simulink model "TGB_V0000"  (R2016b)
settings: Solver=VariableStepAuto  StartTime=0.0  StopTime=350  RelTol=1e-3
values from neighbouring files (symbols this model uses):
  h = 30    [AutoPID.m]
  K = data.Data(len)/100    [AutoPID.m]
  Kp = 0.6*Kc    (= 0.48762365543)    [AutoPID.m]
  Malha = 1    [AutoPID.m]
  N = 1    [AutoPID.m]
  T = (10*wn)/2*pi    [AutoPID.m]
  T_PID = 1    [AutoPID.m]
  tau = (3/2)*(t2-t1)    [AutoPID.m]
  Td = Tc*0.125    (= 41.8060200669)    [AutoPID.m]
  theta = t2-tau    [AutoPID.m]
  Ti = Tc*0.5    (= 167.224080268)    [AutoPID.m]
  TypeControler = 1    [AutoPID.m]
  TypeOutput = 1    [AutoPID.m]
undefined symbols (not defined in the file or in its folder): DiscIntNeverNeededParam
libraries: simulink x2
settings Model: Creator=Workstation - LFC  LastModifiedBy=Gpiaia
settings DataIOCC: SaveOutput=off  SaveTime=off
settings OptimizationCC: DefaultParameterBehavior=Inlined  UseDivisionForNetSlopeComputation=on  UseFloatMulNetSlope=on  InlineInvariantSignals=on  PassReuseOutputArgsAs=Individual arguments  ZeroExternalMemoryAtStartup=off  ZeroInternalMemoryAtStartup=off  NoFixptDivByZeroProtection=on  EfficientFloat2IntCast=on  LifeSpan=1
settings DebuggingCC: ParameterTunabilityLossMsg=error  SFExecutionAtInitializationDiag=none
settings HardwareCC: ProdBitPerLong=64  ProdHWDeviceType=Intel->x86-64 (Linux 64)
settings RTWCC: SystemTargetFile=ert.tlc  TemplateMakefile=ert_default_tmf  Description=Embedded Coder  GenerateReport=on  IncludeHyperlinkInReport=on  LaunchReport=on  GenerateTraceInfo=on  GenerateTraceReport=on  GenerateTraceReportSl=on  GenerateTraceReportSf=on  GenerateTraceReportEml=on  GenerateCodeMetricsReport=on
settings CodeAppCC: ForceParamTrailComments=on  IgnoreCustomStorageClasses=off  OperatorAnnotations=on  SimulinkDataObjDesc=on  SFDataObjDesc=on  MATLABFcnDesc=on  CustomSymbolStrGlobalVar=rt$N$M  CustomSymbolStrType=$N$M  CustomSymbolStrFcn=$N$M$F  CustomSymbolStrMacro=$N$M  InsertBlockDesc=on  MATLABSourceComments=on
settings ERTTargetCC: TargetLangStandard=C99 (ISO)  GenerateSampleERTMain=on  CombineSignalStateStructs=on  SupportComplex=off  SupportNonInlinedSFcns=on  InlinedParameterPlacement=NonHierarchical  ERTCustomFileTemplate=example_file_process.tlc  ERTFilePackagingFormat=CompactWithDataFile

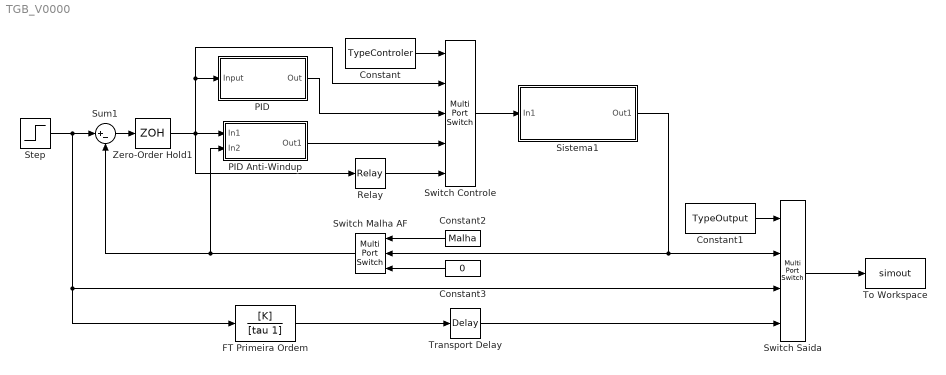
== system TGB_V0000 ==
  Constant : Constant  Value=TypeControler
  Constant1 : Constant  Value=TypeOutput
  Constant2 : Constant  Value=Malha
  Constant3 : Constant  Value=0
  FT Primeira Ordem : TransferFcn  Numerator=[K]  Denominator=[tau 1]
  PID : Subsystem
  PID Anti-Windup : Subsystem
  Relay : Relay  OnSwitchValue=+h  OffSwitchValue=-h  OnOutputValue=+h  OffOutputValue=-h
  Sistema1 : Subsystem
      mask help: Simulink:masks:GenSFuncDesc_MD
      mask Help: eval('feval(''rtwprivate'',''rtwhelpview'',''rtw_sfcn_block'')');
  Step : Step  Time=0  After=100  SampleTime=0
  Sum1 : Sum  Inputs=|+-
  Switch Controle : MultiPortSwitch  Inputs=4  SaturateOnIntegerOverflow=on
  Switch Malha AF : MultiPortSwitch  Inputs=2  SaturateOnIntegerOverflow=on
  Switch Saida : MultiPortSwitch  SaturateOnIntegerOverflow=on
  To Workspace : ToWorkspace  VariableName=simout  SaveFormat=Timeseries  SampleTime=-1
  Transport Delay : TransportDelay  DelayTime=theta
  Zero-Order Hold1 : ZeroOrderHold  SampleTime=T
  wires:
  Sum1/1 -> Zero-Order Hold1/1
  Step/1 -> Switch Saida/3, FT Primeira Ordem/1, Sum1/1
  FT Primeira Ordem/1 -> Transport Delay/1
  Sistema1/1(Out1) -> Switch Malha AF/2, Switch Saida/2
  Zero-Order Hold1/1 -> Switch Controle/2, PID/1(Input), Relay/1, PID Anti-Windup/1(In1)
  PID Anti-Windup/1(Out1) -> Switch Controle/4
  PID/1(Out) -> Switch Controle/3
  Transport Delay/1 -> Switch Saida/4
  Switch Saida/1 -> To Workspace/1
  Constant/1 -> Switch Controle/1
  Constant1/1 -> Switch Saida/1
  Switch Malha AF/1 -> Sum1/2, PID Anti-Windup/2(In2)
  Constant2/1 -> Switch Malha AF/1
  Constant3/1 -> Switch Malha AF/3
  Switch Controle/1 -> Sistema1/1(In1)
  Relay/1 -> Switch Controle/5

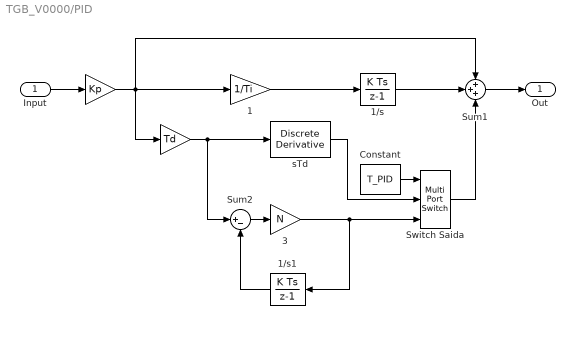
== system TGB_V0000/PID ==
  Input : Inport
  " " : Gain  Gain=Kp
  " " : Gain  Gain=Td
  " 1" : Gain  Gain=1/Ti
  " 3" : Gain  Gain=N
  1/s : DiscreteIntegrator  gainval=1  InitialConditionSetting=State (most efficient)  SampleTime=T  ICPrevOutput=DiscIntNeverNeededParam  ICPrevScaledInput=DiscIntNeverNeededParam
  1/s1 : DiscreteIntegrator  gainval=1  InitialConditionSetting=State (most efficient)  SampleTime=T  ICPrevOutput=DiscIntNeverNeededParam  ICPrevScaledInput=DiscIntNeverNeededParam
  Constant : Constant  Value=T_PID
  Sum1 : Sum  Inputs=+++
  Sum2 : Sum  Inputs=|+-
  Switch Saida : MultiPortSwitch  Inputs=2  SaturateOnIntegerOverflow=on
  sTd : simulink/Discrete/Discrete Derivative  gainval=1  ICPrevScaledInput=0.0  OutMin=[]  OutMax=[]  OutDataType=fixdt(1, 16)  OutScaling=2^-10  DoSatur=off
  Out : Outport
  wires:
  Sum1/1 -> Out/1
  Input/1 -> " "/1
  1/s/1 -> Sum1/2
  " "/1 -> " "/1, " 1"/1, Sum1/1
  " 1"/1 -> 1/s/1
  " "/1 -> sTd/1, Sum2/1
  Switch Saida/1 -> Sum1/3
  Sum2/1 -> " 3"/1
  sTd/1 -> Switch Saida/2
  Constant/1 -> Switch Saida/1
  " 3"/1 -> 1/s1/1, Switch Saida/3
  1/s1/1 -> Sum2/2

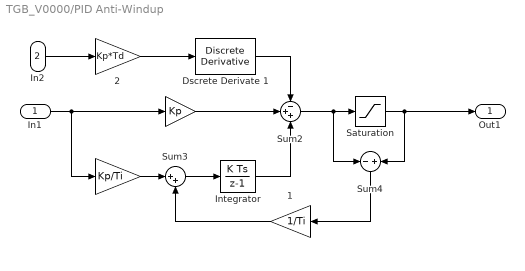
== system TGB_V0000/PID Anti-Windup ==
  In1 : Inport
  In2 : Inport  Port=2
  " " : Gain  Gain=Kp
  "  " : Gain  Gain=Kp/Ti
  "  1" : Gain  Gain=1/Ti
  "  2" : Gain  Gain=Kp*Td
  Dscrete Derivate 1 : simulink/Discrete/Discrete Derivative  gainval=1  ICPrevScaledInput=0.0  OutMin=[]  OutMax=[]  OutDataType=fixdt(1, 16)  OutScaling=2^-10  DoSatur=off
  Integrator : DiscreteIntegrator  gainval=1  InitialConditionSetting=State (most efficient)  SampleTime=T  ICPrevOutput=DiscIntNeverNeededParam  ICPrevScaledInput=DiscIntNeverNeededParam
  Saturation : Saturate  UpperLimit=90  LowerLimit=-90
  Sum2 : Sum  Inputs=-++
  Sum3 : Sum  Inputs=|++
  Sum4 : Sum  Inputs=-+
  Out1 : Outport
  wires:
  Integrator/1 -> Sum2/3
  Sum3/1 -> Integrator/1
  "  1"/1 -> Sum3/2
  "  "/1 -> Sum3/1
  Saturation/1 -> Out1/1, Sum4/2
  Sum4/1 -> "  1"/1
  Sum2/1 -> Saturation/1, Sum4/1
  Dscrete Derivate 1/1 -> Sum2/1
  In1/1 -> " "/1, "  "/1
  " "/1 -> Sum2/2
  "  2"/1 -> Dscrete Derivate 1/1
  In2/1 -> "  2"/1

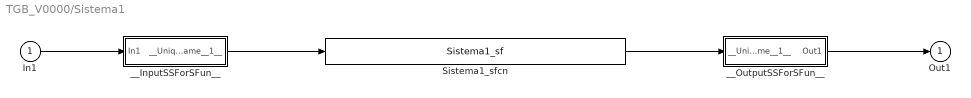
== system TGB_V0000/Sistema1 ==
  In1 : Inport
  Sistema1_sfcn : S-Function  FunctionName=Sistema1_sf  SFunctionModules=""  SFunctionDeploymentMode=off  EnableBusSupport=off  mask{rtw_sf_name=Sistema1_sf, showVar=off}
      mask prompts: rtw_sf_name "Simulink:masks:GenSFuncName_MP"; showVar "Simulink:masks:GenSFuncShowModuleList_MP"
      mask help: Simulink:masks:GenSFuncDesc_MD
      mask init:
      | displist = '';
      | if ~strcmp(get_param(gcb, 'FunctionName'), rtw_sf_name);
      |   set_param(gcb, 'FunctionName', rtw_sf_name);
      | end
      | % Check if we are generating code
      | rtw_mode = false;
      | if strcmpi(get_param(bdroot(gcb),'SimulationStatus'),'Initializing')
      | 	rtw_mode = strcmpi(get_param(bdroot(gcb),'BuildingRTWCode'),'on') && ...
      | 		~strcmpi(get_param(bdroot(gcb),'TargetStyle'),'SimulationTarget');
      | end
      | if showVar || rtw_mode
      | 	if exist('rtwsfunc') == 2 | exist('rtwsfunc') == 6
      | 		tmplist = rtwsfunc(rtw_sf_name,gcb);
      | 		tmplist = DAStudio.message('Simulink:masks:GenSFuncListOfModules_IC', tmplist);
      | 	elseif showVar
      | 		tmplist1 = DAStudio.message('Simulink:masks:GenSFuncListOfModules_IC', '');
      |         tmplist2 = DAStudio.message('Simulink:masks:GenSFuncNotLicensed_IC');
      |         tmplist = [tmplist1 tmplist2];
      |  	end
      | end
      | if showVar
      |   displist = tmplist;
      | end
      settings: CopyFcn=|
      | if ~strcmp(get_param(gcb,'Linkstatus'),'none') && ...
      | ~strcmp(get_param(gcb,'Linkstatus'),'implicit')
      |   set_param(gcb,'LinkStatus','none');
      | end
      mask Help: eval('feval(''rtwprivate'',''rtwhelpview'',''rtw_sfcn_block'')');
      mask Display:
      | port_label('input',1,'In1');
      | port_label('output',1,'Out1');
  __InputSSForSFun__ : Subsystem
  __OutputSSForSFun__ : Subsystem
  Out1 : Outport
  wires:
  In1/1 -> __InputSSForSFun__/1(In1)
  __InputSSForSFun__/1(__UniqueOutportName__1__) -> Sistema1_sfcn/1
  Sistema1_sfcn/1 -> __OutputSSForSFun__/1(__UniqueInportName__1__)
  __OutputSSForSFun__/1(Out1) -> Out1/1

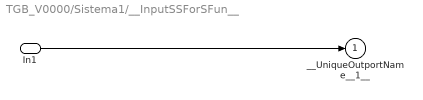
== system TGB_V0000/Sistema1/__InputSSForSFun__ ==
  In1 : Inport
  __UniqueOutportName__1__ : Outport
  wires:
  In1/1 -> __UniqueOutportName__1__/1

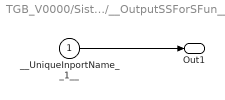
== system TGB_V0000/Sistema1/__OutputSSForSFun__ ==
  __UniqueInportName__1__ : Inport
  Out1 : Outport
  wires:
  __UniqueInportName__1__/1 -> Out1/1
